simulink model "schemat"  (R2022b)
settings: Solver=FixedStepAuto  StartTime=0.0  StopTime=20.0  FixedStep=0.01  RelTol=1e-3
values from neighbouring files (symbols this model uses):
  dt = 0.1    [zad1.m]    (also in zad2.m)
  kp = 2    [zad2.m]
undefined symbols (not defined in the file or in its folder): dend, DiscIntNeverNeededParam, num
settings Model: Creator=asialalala  LastModifiedBy=asialalala

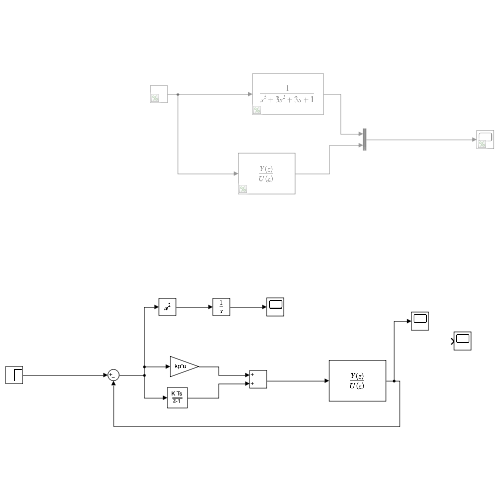
[thumbnail: Simulink's stored preview of the top-level diagram]
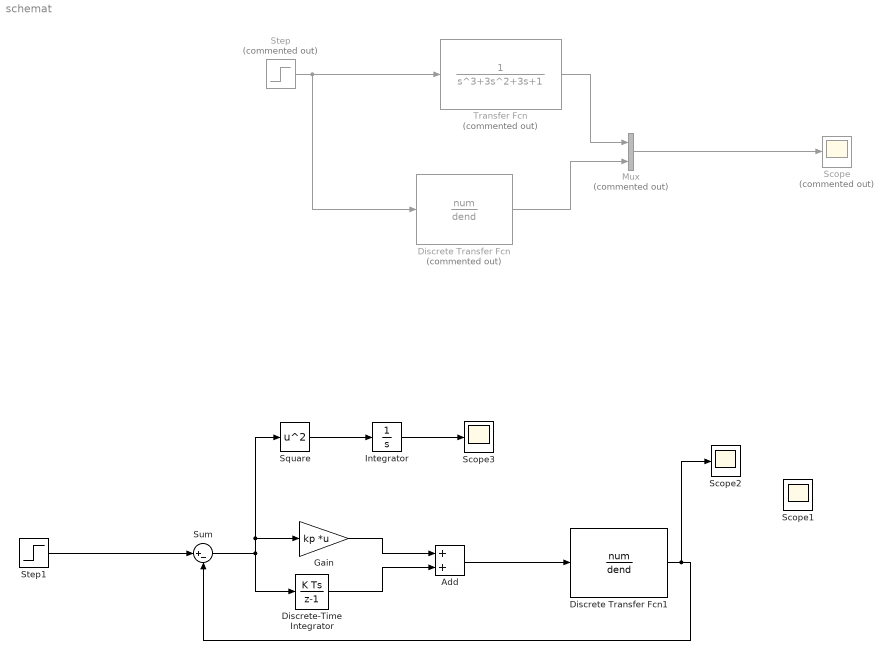
== system schemat ==
  Add : Sum
  Discrete Transfer Fcn : DiscreteTransferFcn  Commented=on  Numerator=num  Denominator=dend  SampleTime=dt
  Discrete Transfer Fcn1 : DiscreteTransferFcn  Numerator=num  Denominator=dend  SampleTime=dt
  Discrete-Time Integrator : DiscreteIntegrator  gainval=ki  SampleTime=dt  ICPrevOutput=DiscIntNeverNeededParam  ICPrevScaledInput=DiscIntNeverNeededParam
  Gain : Gain  Gain=kp  Multiplication=Matrix(K*u)
  Integrator : Integrator
  Mux : Mux  Commented=on  Inputs=2
  Scope : Scope  Commented=on
  Scope1 : Scope
  Scope2 : Scope
  Scope3 : Scope
  Square : Math  Operator=square
  Step : Step  Commented=on  SampleTime=0
  Step1 : Step  SampleTime=0
  Sum : Sum  Inputs=|+-
  Transfer Fcn : TransferFcn  Commented=on  Denominator=[1 3 3 1]
  wires:
  Step/1 -> Discrete Transfer Fcn/1, Transfer Fcn/1
  Mux/1 -> Scope/1
  Transfer Fcn/1 -> Mux/1
  Discrete Transfer Fcn/1 -> Mux/2
  Step1/1 -> Sum/1
  Sum/1 -> Discrete-Time Integrator/1, Square/1, Gain/1
  Discrete Transfer Fcn1/1 -> Scope2/1, Sum/2
  Add/1 -> Discrete Transfer Fcn1/1
  Gain/1 -> Add/1
  Discrete-Time Integrator/1 -> Add/2
  Square/1 -> Integrator/1
  Integrator/1 -> Scope3/1
